simulink model "Boat_Model"  (R2017a)
settings: Solver=VariableStepAuto  StartTime=0.0  StopTime=10.0  RelTol=1e-3
settings Model: Creator=John  LastModifiedBy=John

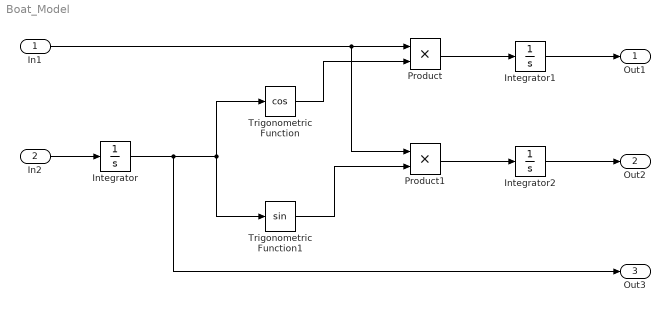
== system Boat_Model ==
  In1 : Inport
  In2 : Inport  Port=2
  Integrator : Integrator
  Integrator1 : Integrator
  Integrator2 : Integrator
  Product : Product
  Product1 : Product
  Trigonometric Function : Trigonometry  Operator=cos
  Trigonometric Function1 : Trigonometry
  Out1 : Outport
  Out2 : Outport  Port=2
  Out3 : Outport  Port=3
  wires:
  In1/1 -> Product1/1, Product/1
  In2/1 -> Integrator/1
  Product/1 -> Integrator1/1
  Product1/1 -> Integrator2/1
  Integrator2/1 -> Out2/1
  Integrator1/1 -> Out1/1
  Trigonometric Function/1 -> Product/2
  Trigonometric Function1/1 -> Product1/2
  Integrator/1 -> Out3/1, Trigonometric Function1/1, Trigonometric Function/1
